simulink model "controller"  (R2025b)
settings: Solver=VariableStepAuto  StartTime=0.0  StopTime=10.0  RelTol=1e-3
values from neighbouring files (symbols this model uses):
  A = [0 1 0 0 ... (first row only)    [untitled2.m]    (also in untitled3.m)
  Aref = 0.8    [untitled3.m]
  B = [0; 0; 0; 1/m2]    [untitled2.m]    (also in untitled3.m = [0;1/m1;0;0])
  c1 = 2    [untitled2.m]    (also in untitled3.m)
  c2 = 5    [untitled2.m]    (also in untitled3.m)
  k1 = 4    [untitled2.m]    (also in untitled3.m)
  k2 = 12    [untitled2.m]    (also in untitled3.m)
  Kd = 35    [untitled3.m]
  Ki = 10    [untitled3.m]
  Kp = 120    [untitled3.m]
  m1 = 3    [untitled2.m]    (also in untitled3.m)
  w = 2*pi*1    (= 6.28318530718)    [untitled3.m]
settings Model: Creator=Abhi  LastModifiedBy=Abhi

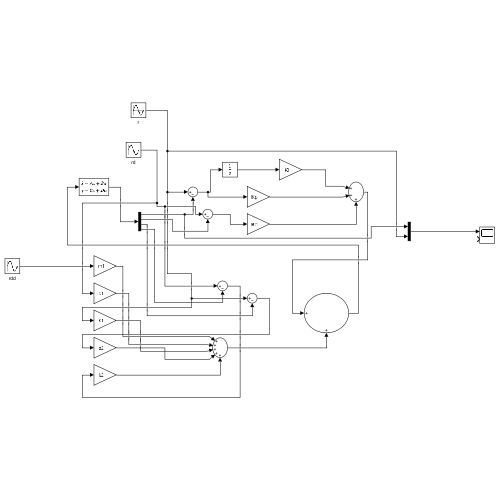
[thumbnail: Simulink's stored preview of the top-level diagram]
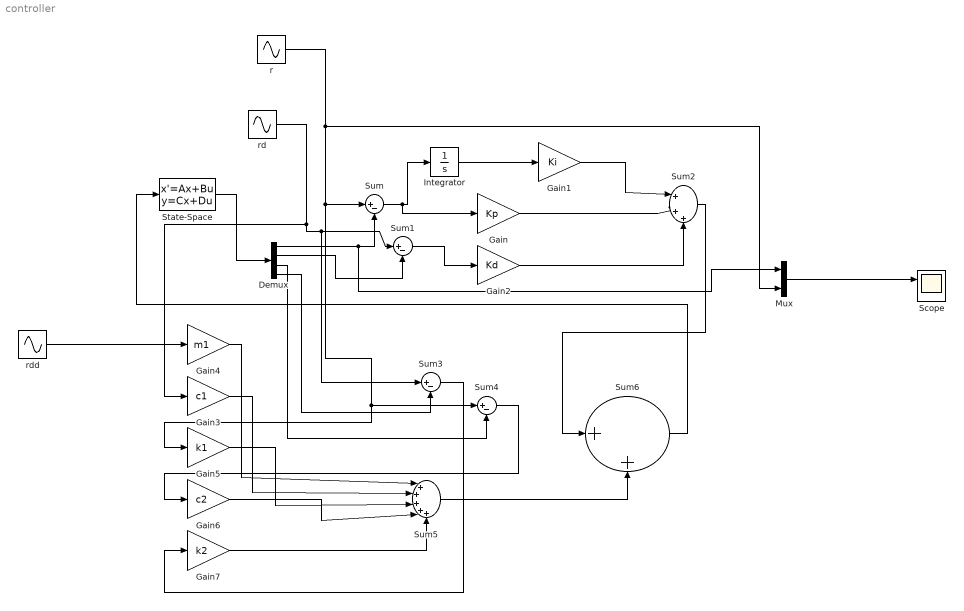
== system controller ==
  Demux : Demux
  Gain : Gain  Gain=Kp
  Gain1 : Gain  Gain=Ki
  Gain2 : Gain  Gain=Kd
  Gain3 : Gain  Gain=c1
  Gain4 : Gain  Gain=m1
  Gain5 : Gain  Gain=k1
  Gain6 : Gain  Gain=c2
  Gain7 : Gain  Gain=k2
  Integrator : Integrator
  Mux : Mux  Inputs=2
  Scope : Scope  NumInputPorts=2
      settings: ActiveDisplayYMinimum=-1.16819116268996  ActiveDisplayYMaximum=1.1667330676781473
  State-Space : StateSpace  A=A  B=B  C=eye(4)  D=zeros(4,1)  InitialCondition=[0.3 0.01 0 0]'
  Sum{,1,3..4} (4 alike) : Sum  Inputs=|+-
  Sum2 : Sum  Inputs=|+++
  Sum5 : Sum  Inputs=|+++++
  Sum6 : Sum  Inputs=|++
  r : Sin  Amplitude=Aref  Frequency=w  SampleTime=0
  rd : Sin  Amplitude=Aref*w  Frequency=w  Phase=pi/2  SampleTime=0
  rdd : Sin  Amplitude=Aref*w*w  Frequency=w  Phase=pi  SampleTime=0
  wires:
  State-Space/1 -> Demux/1
  Demux/1 -> Mux/1, Sum/2
  r/1 -> Mux/2, Gain5/1, Sum4/1, Sum/1
  Sum/1 -> Gain/1, Integrator/1
  Demux/2 -> Sum1/2
  rd/1 -> Gain3/1, Sum3/1, Sum1/1
  Integrator/1 -> Gain1/1
  Sum1/1 -> Gain2/1
  Gain1/1 -> Sum2/1
  Gain/1 -> Sum2/2
  Gain2/1 -> Sum2/3
  Demux/4 -> Sum3/2
  Demux/3 -> Sum4/2
  rdd/1 -> Gain4/1
  Sum3/1 -> Gain7/1
  Sum4/1 -> Gain6/1
  Gain4/1 -> Sum5/1
  Gain3/1 -> Sum5/2
  Gain5/1 -> Sum5/3
  Gain6/1 -> Sum5/4
  Gain7/1 -> Sum5/5
  Sum2/1 -> Sum6/1
  Sum5/1 -> Sum6/2
  Sum6/1 -> State-Space/1
  Mux/1 -> Scope/1
